simulink model "PWM_SIMULINK"  (R2014a)
settings: Solver=ode45  StartTime=0.0  StopTime=10.0  RelTol=1e-3
libraries: simulink x1
settings Model: Creator=User  LastModifiedBy=admin
settings DebuggingCC: UnderspecifiedInitializationDetection=Classic  SolverPrmCheckMsg=none  StateNameClashWarn=warning

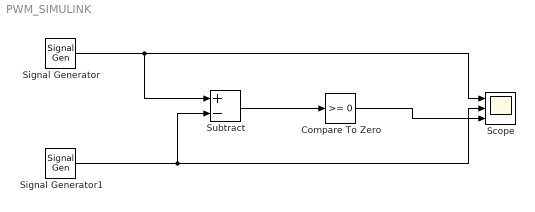
== system PWM_SIMULINK ==
  Compare To Zero : simulink/Logic and Bit Operations/Compare To Zero  relop=>=  OutDataTypeStr=uint8
  Scope : Scope  NumInputPorts=3
      settings: YMin=-5~-5~-5  YMax=5~5~5
  Signal Generator : SignalGenerator  Units=rad/sec
  Signal Generator1 : SignalGenerator  WaveForm=sawtooth  Frequency=10  Units=rad/sec
  Subtract : Sum  Inputs=+-
  wires:
  Signal Generator/1 -> Scope/1, Subtract/1
  Signal Generator1/1 -> Scope/2, Subtract/2
  Subtract/1 -> Compare To Zero/1
  Compare To Zero/1 -> Scope/3
